simulink model "untitled"  (R2023a)
settings: Solver=VariableStepAuto  StartTime=0.0  StopTime=10.0  RelTol=1e-3
undefined symbols (not defined in the file): S
libraries: simrfV2util1 x3, simrfV2elements x2, simrfV2sources1 x1, simrfV2junction1 x1, dspstat3 x1
settings Model: Creator=ania  LastModifiedBy=ania

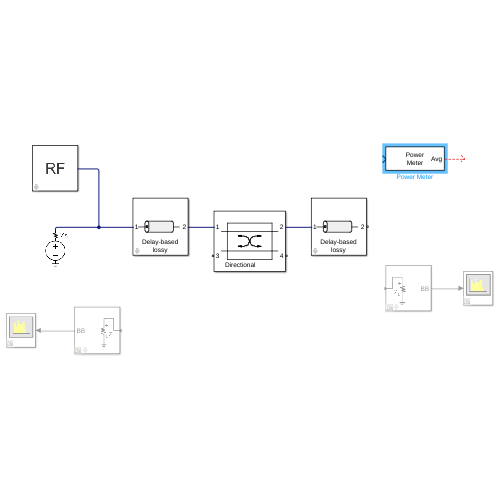
[thumbnail: Simulink's stored preview of the top-level diagram]
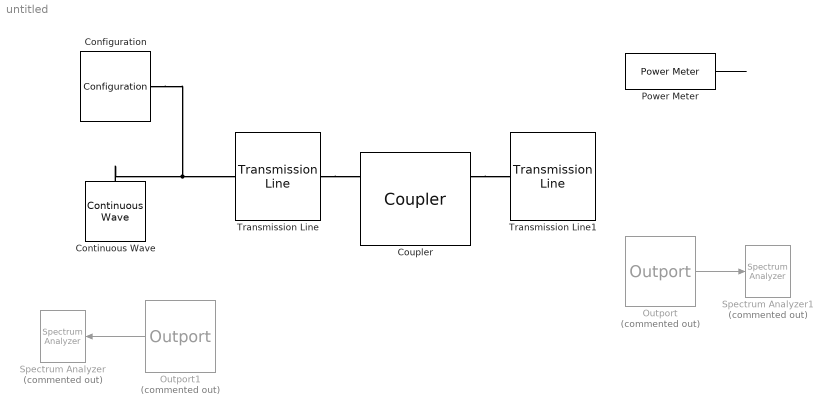
== system untitled ==
  Configuration : simrfV2util1/Configuration  AutoFreq=on  Tones=[1.8] GHz  Harmonics=[7]  NormalizeCarrierPower=on  SolverType=Auto  UseCCode=on  StepSize=1e-6 s  AddNoise=off  defaultRNG=on  Seed=0  Temperature=290.0 K  SolverDelFlag=0  AbsTol=1e-6  RelTol=1e-3  MaxIter=10  ErrorEstimationType=2-norm over all variables  EnableInterpFilter=off  HiddenFIRfilterControllerParam=on  SmallSignalApprox=off  AllSimFreqs=on  SimFreqs=[] Hz  SimFreqsInternal=[]  SamplesPerFrame=1
  Continuous Wave : simrfV2sources1/Continuous Wave  CWSourceType=Power  Z0=50  IVoltage=0 V  ICurrent=0 A  MagPower=-6 dBm  QVoltage=0 V  QCurrent=0 A  AnglePower=0  CarrierFreq=1.8 GHz  AddPhaseNoise=off  PhaseNoiseOffset=1  PhaseNoiseLevel=-Inf  AutoImpulseLength=on  ImpulseLength=1e-10 s  InternalGrounding=on
  Coupler : simrfV2junction1/Coupler  classname=couplers  DataSource=Network-parameters  NumPorts=4  DeviceCirculator=Circulator clockwise  DeviceDivider=T power divider  DeviceCoupler=Directional coupler  Paramtype=S-parameters  Sparam=[0 0 1; 1 0 0; 0 1 0]  SparamFreq=1e9 Hz  SparamZ0=50  Phase12=0  Phase33=0  Alpha=0  NumberDividerOutports=2  Coupling=3  Directivity=inf  InsertionLoss=inf  ReturnLoss=inf  InternalGrounding=on  SparamRepresentation=Frequency domain  FitOpt=Share all poles  FitTol=-40  MaxPoles=48
  Outport : simrfV2util1/Outport  Commented=on  SensorType=Power  OutputFormat=Complex Baseband  CarrierFreq=1.8 GHz  ZL=1  InternalGrounding=on  StepSize=1e-6 s  AutoStep=on  HalfPolyphaseLength=12
  Outport1 : simrfV2util1/Outport  Commented=on  SensorType=Power  OutputFormat=Complex Baseband  CarrierFreq=1.8 GHz  ZL=1  InternalGrounding=on  StepSize=1e-6 s  AutoStep=on  HalfPolyphaseLength=12
  Power Meter : dspstat3/Power Meter  Measurement=Average power  ReferenceLoad=50  OutputPowerUnits=dBm  WindowLength=256  OverlapLength=255  AllowArbitraryInputLength=off  ComputeCCDF=off  PowerRange=50  PowerResolution=0.1  CCDFOutput=Relative power (dB above average power)  ProbabilityVector=[ 10; 1; 0.1; 0.01; 0.001; 0.0001 ]  RelativePowerVector=[ 0; 3; 6; 9; 12 ]  ResetPort=off  SimulateUsing=Code generation
  Spectrum Analyzer : SpectrumAnalyzer  Commented=on  WindowPosition=[950.000000,424.000000,800.000000,500.000000,]  Visible=on  ScopeFrameLocation=window  YLimits=[-264.96029562,-207.53619117]  ColorLimits=[-80 20]
  Spectrum Analyzer1 : SpectrumAnalyzer  Commented=on  WindowPosition=[560.000000,290.000000,800.000000,500.000000,]  ScopeFrameLocation=window  YLimits=[-293.5657205,-228.05331379]  ColorLimits=[-80 20]
  Transmission Line : simrfV2elements/Transmission Line  classname=xline  Model_type=Delay-based and lossy  ConductorBacked=off  StructureMicrostrip=Standard  Parameterization=By characteristic impedance and capacitance  TransDelay=4.7e-9 s  CharImped=50 Ohm  Resistance=0 Ohm/m  Inductance=235e-9 H/m  Capacitance=94e-12 F/m  Conductance=5e-6 S/m  LineLength=15 mm  NumSegments=10  InternalGrounding=on  OuterRadius=2.57 mm  InnerRadius=0.725 mm  MuR=1  EpsilonR=2.2  LossTangent=0  SigmaCond=inf S/m  StubMode=Not a stub  Termination=Open  ConductorWidth=0.6 mm  SlotWidth=0.2 mm  Height=0.635 mm  Height_inv=0.635 mm  Height_spd=0.3175 mm  Height_emb=1.37 mm  StripHeight=0.635 mm  Thickness=5 um  SWidth=0.6 mm  Radius=0.67 mm  Separation=1.62 mm  PWidth=5 mm  PSeparation=1 mm  PV=299792458  Loss=0  SourceFreq=User-specified  PlotFreq=[1e9:1e6:3e9] Hz  PlotType=X-Y plane  YParam1=S(1,1)  YFormat1=Magnitude (dB)  YParam2=S(2,2)  YFormat2=Magnitude (dB)  YOption=Linear  XOption=Linear  FitOpt=Share all poles  FitTol=-40  MaxPoles=48  SparamRepresentation=Frequency domain  Freq=1e9 Hz  Interp_type=Linear  AutoImpulseLength=off  ImpulseLength=0 s  MagModeling=off
  Transmission Line1 : simrfV2elements/Transmission Line  classname=xline  Model_type=Delay-based and lossy  ConductorBacked=off  StructureMicrostrip=Standard  Parameterization=By characteristic impedance and capacitance  TransDelay=4.7e-9 s  CharImped=50 Ohm  Resistance=0 Ohm/m  Inductance=235e-9 H/m  Capacitance=94e-12 F/m  Conductance=5e-6 S/m  LineLength=15 mm  NumSegments=10  InternalGrounding=on  OuterRadius=2.57 mm  InnerRadius=0.725 mm  MuR=1  EpsilonR=2.2  LossTangent=0  SigmaCond=inf S/m  StubMode=Not a stub  Termination=Open  ConductorWidth=0.6 mm  SlotWidth=0.2 mm  Height=0.635 mm  Height_inv=0.635 mm  Height_spd=0.3175 mm  Height_emb=1.37 mm  StripHeight=0.635 mm  Thickness=5 um  SWidth=0.6 mm  Radius=0.67 mm  Separation=1.62 mm  PWidth=5 mm  PSeparation=1 mm  PV=299792458  Loss=0  SourceFreq=User-specified  PlotFreq=[1e9:1e6:3e9] Hz  PlotType=X-Y plane  YParam1=S(1,1)  YFormat1=Magnitude (dB)  YParam2=S(2,2)  YFormat2=Magnitude (dB)  YOption=Linear  XOption=Linear  FitOpt=Share all poles  FitTol=-40  MaxPoles=48  SparamRepresentation=Frequency domain  Freq=1e9 Hz  Interp_type=Linear  AutoImpulseLength=off  ImpulseLength=0 s  MagModeling=off
  wires:
  Outport1/1 -> Spectrum Analyzer/1
  Outport/1 -> Spectrum Analyzer1/1
  Power Meter/1 -> ?
  connections:
  Configuration/LConn1 -- Continuous Wave/LConn1 -- Transmission Line/LConn1
  Transmission Line/RConn1 -- Coupler/LConn1
  Coupler/RConn1 -- Transmission Line1/LConn1
